simulink model "StepMotor"  (R2021b)
settings: Solver=FixedStepAuto  StartTime=0.0  StopTime=inf  RelTol=1e-3  EnableMultiTasking=on
model workspace (MAT data in the model file):
  freq = 490.2
values from neighbouring files (symbols this model uses):
  n_step = Ctrl_freq/PWM_freq    (= 100)    [para_step.m]
  Tc = 1/Ctrl_freq    (= 0.0002)    [para_step.m]
  width_step = n_step/2    (= 50)    [para_step.m]
libraries: arduinolib x5
settings Model: ExtModeTrigDuration=2  Creator=yolee  LastModifiedBy=yolee
settings SolverCC: AutoInsertRateTranBlk=on
settings OptimizationCC: EnhancedBackFolding=on  PassReuseOutputArgsAs=Individual arguments  ZeroExternalMemoryAtStartup=off  ZeroInternalMemoryAtStartup=off  MaxStackSize=64  OptimizeBlockOrder=speed  DifferentSizesBufferReuse=on  OptimizationCustomize=off  EfficientTunableParamExpr=on
settings DebuggingCC: ParameterTunabilityLossMsg=error
settings HardwareCC: ProdBitPerInt=16  ProdBitPerPointer=16  ProdBitPerSizeT=16  ProdBitPerPtrDiffT=16  ProdLargestAtomicFloat=None  ProdWordSize=8  ProdHWDeviceType=Atmel->AVR
settings SFSimCC: MATLABDynamicMemAlloc=off
settings RTWCC: Description=Embedded Coder  SystemTargetFile=ert.tlc  HardwareBoard=Arduino Mega 2560  TemplateMakefile=ert_default_tmf  Toolchain=Arduino AVR  BuildConfiguration=Faster Runs
settings CodeAppCC: ForceParamTrailComments=on  IgnoreCustomStorageClasses=off  OperatorAnnotations=on  SimulinkDataObjDesc=on  SFDataObjDesc=on  InsertBlockDesc=on
settings ERTTargetCC: SupportContinuousTime=on  SupportVariableSizeSignals=on  ExtModeTransport=3  ExtModeStaticAlloc=on  ExtModeStaticAllocSize=2048  ExtModeMexFile=ext_xcp  ExtModeIntrfLevel=Level2 - Open

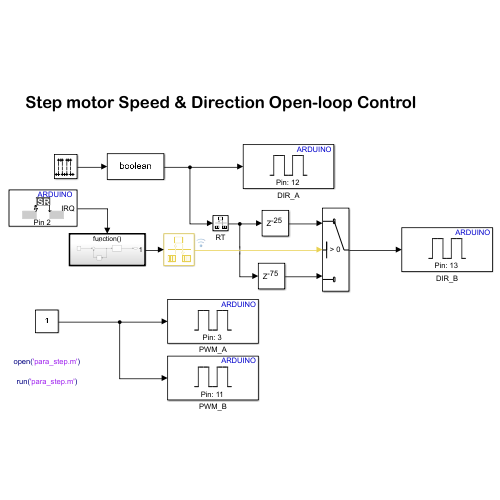
[thumbnail: Simulink's stored preview of the top-level diagram]
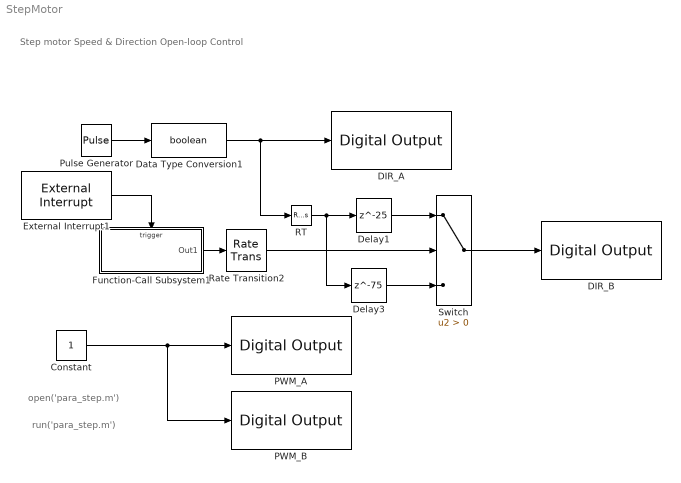
== system StepMotor ==
  note: open('para_step.m')
  note: run('para_step.m')
  note: Step motor Speed & Direction Open-loop Control
  Constant : Constant
  DIR_A : arduinolib/Digital Output  pinNumber=12  Direction=output  blockPlatform=arduino
  DIR_B : arduinolib/Digital Output  pinNumber=13  Direction=output  blockPlatform=arduino
  Data Type Conversion1 : DataTypeConversion  OutDataTypeStr=boolean
  Delay1 : Delay  DelayLength=25  InitialCondition=0  SampleTime=Tc
  Delay3 : Delay  DelayLength=75  InitialCondition=0  SampleTime=Tc
  External Interrupt1 : arduinolib/External Interrupt  Pin=2  PullUp=off  Mode=FALLING  InterruptSimulationInput=off
      settings: SourceProductBaseCode=ARDUINO
  Function-Call Subsystem1 : Subsystem  TreatAsAtomicUnit=on
  PWM_A : arduinolib/Digital Output  pinNumber=3  Direction=output  blockPlatform=arduino
  PWM_B : arduinolib/Digital Output  pinNumber=11  Direction=output  blockPlatform=arduino
  Pulse Generator : DiscretePulseGenerator  Period=n_step  PulseWidth=width_step  SampleTime=Tc
  RT : RateTransition  OutPortSampleTime=Tc
  Rate Transition2 : RateTransition  Deterministic=off  OutPortSampleTime=Tc
  Switch : Switch  Criteria=u2 > Threshold
  wires:
  Pulse Generator/1 -> Data Type Conversion1/1
  Data Type Conversion1/1 -> RT/1, DIR_A/1
  Constant/1 -> PWM_B/1, PWM_A/1
  Rate Transition2/1 -> Switch/2
  Delay1/1 -> Switch/1
  Switch/1 -> DIR_B/1
  External Interrupt1/1 -> Function-Call Subsystem1/Trigger
  Function-Call Subsystem1/1(Out1) -> Rate Transition2/1
  RT/1 -> Delay3/1, Delay1/1
  Delay3/1 -> Switch/3

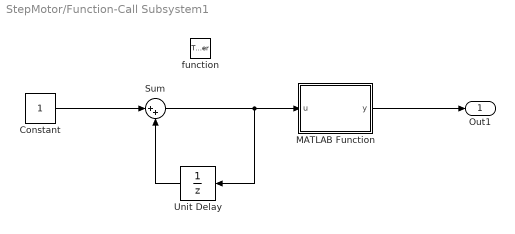
== system StepMotor/Function-Call Subsystem1 ==
  function : TriggerPort  TriggerType=function-call  VariantControl=(inherit)
  Constant : Constant
  MATLAB Function : MATLAB Function  TreatAsAtomicUnit=on
  Sum : Sum  Inputs=|++
  Unit Delay : UnitDelay  SampleTime=-1  HasFrameUpgradeWarning=on
  Out1 : Outport
  wires:
  Constant/1 -> Sum/1
  Unit Delay/1 -> Sum/2
  Sum/1 -> Unit Delay/1, MATLAB Function/1(u)
  MATLAB Function/1(y) -> Out1/1

== matlab function StepMotor/Function-Call Subsystem1/MATLAB Function ==
  data: u input; y output
function y = fcn(u)
 rem = mod(u,2);
 if rem == 0
     y=0;
 else
     y=1;
 end

 if u > 100
     u = 1;
 end
